simulink model "Capture_NDI"  (R2023b)
settings: Solver=FixedStepAuto  StartTime=0.0  StopTime=3500  RelTol=1e-3
values from neighbouring files (symbols this model uses):
  dim_q = robot_post_sim.n_q    [init_control_test.m]
  dim_r = robot_post_sim.dimensions.dim_r    [init_control_test.m]
  q00 = [0;0;0;1;zeros(3,1)]    [init_control_test.m]
  qm0 = q_init    [init_control_test.m]
  robot_unc_post = get_robot_unc(robot_post_sim,robot_post,E_inertia_max,E_mass_max,E_mode_max,E_mass_target_max,E_inertia_target_max)    [init_control_test.m]
  robot_unc_pre = get_robot_unc(robot_pre_sim,robot_pre,E_inertia_max,E_mass_max,E_mode_max,E_mass_target_max,E_inertia_target_max)    [init_control_test.m]
  u0_t_0 = rand(6,1)*1e-4    [init_control_test.m]
  um0 = qdot_init    [init_control_test.m]
undefined symbols (not defined in the file or in its folder): Newton, Raphson, robot_post_sim, robot_pre_sim, target_sim
libraries: SPART_Lib x1
settings Model: Creator=skraiem  LastModifiedBy=skraiem

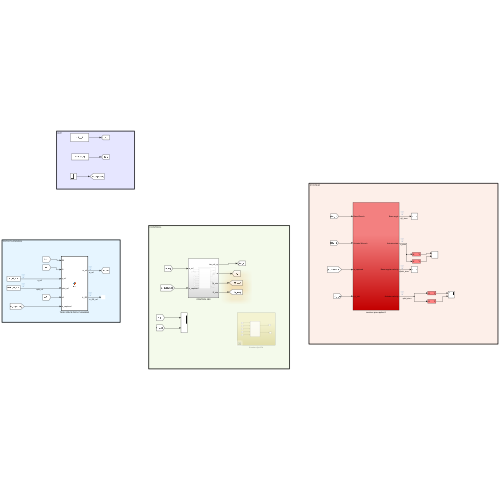
[thumbnail: Simulink's stored preview of the top-level diagram]
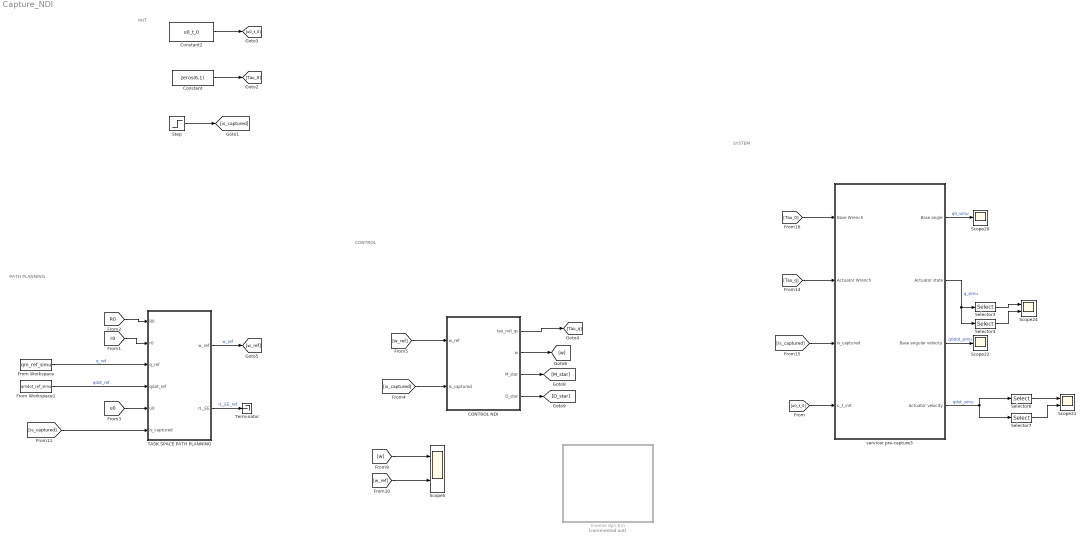
== system Capture_NDI ==
  note: SYSTEM
  note: CONTROL
  note: PATH PLANNING
  note: INIT
  CONTROL NDI : Subsystem
  Constant : Constant  Value=zeros(6,1)
  Constant2 : Constant  Value=u0_t_0
  From Workspace : FromWorkspace  VariableName=qm_ref_simu
  From Workspace1 : FromWorkspace  VariableName=qmdot_ref_simu
  Inverse dyn-Kin : Subsystem  Commented=on
  Scope20 : Scope
  Scope21 : Scope  NumInputPorts=2
  Scope22 : Scope
  Scope24 : Scope  NumInputPorts=2
  Scope5 : Scope  NumInputPorts=2
  Selector3 : Selector  IndexOptions=Index vector (dialog)  Indices=[1:dim_r]  OutputSizes=1
  Selector4 : Selector  IndexOptions=Index vector (dialog)  Indices=[dim_r+1:dim_q]  OutputSizes=1
  Selector6 : Selector  IndexOptions=Index vector (dialog)  Indices=[1:dim_r]  OutputSizes=1
  Selector7 : Selector  IndexOptions=Index vector (dialog)  Indices=[dim_r+1:dim_q]  OutputSizes=1
  Step : Step  Time=2050  SampleTime=0
  TASK SPACE PATH PLANNING : MATLAB Function  TreatAsAtomicUnit=on
  Terminator : Terminator
  servicer pre-capture3 : Subsystem
  wires:
  Step/1 -> [is_captured]
  Constant/1 -> [Tau_0]
  [Tau_0] -> servicer pre-capture3/1(Base Wrench)
  [is_captured] -> servicer pre-capture3/3(is_captured)
  servicer pre-capture3/2(Actuator state) -> Selector3/1, Selector4/1  "q_simu"
  servicer pre-capture3/4(Actuator velocity) -> Selector7/1, Selector6/1  "qdot_simu"
  servicer pre-capture3/3(Base angular velocity) -> Scope22/1  "q0dot_simu"
  servicer pre-capture3/1(Base angle) -> Scope20/1  "q0_simu"
  [u0_t_0] -> servicer pre-capture3/4(u_t_init)
  [Tau_q] -> servicer pre-capture3/2(Actuator Wrench)
  Selector3/1 -> Scope24/1
  Selector4/1 -> Scope24/2
  Selector6/1 -> Scope21/1
  Selector7/1 -> Scope21/2
  Constant2/1 -> [u0_t_0]
  From Workspace/1 -> TASK SPACE PATH PLANNING/3(q_ref)  "q_ref"
  From Workspace1/1 -> TASK SPACE PATH PLANNING/4(qdot_ref)  "qdot_ref"
  [r0] -> TASK SPACE PATH PLANNING/2(r0)
  [R0] -> TASK SPACE PATH PLANNING/1(R0)
  TASK SPACE PATH PLANNING/1(w_ref) -> [w_ref]  "w_ref"
  [u0] -> TASK SPACE PATH PLANNING/5(u0)
  [is_captured] -> CONTROL NDI/2(is_captured)
  CONTROL NDI/2(w) -> [w]
  TASK SPACE PATH PLANNING/2(rL_EE) -> Terminator/1  "rL_EE_ref"
  CONTROL NDI/1(tau_ndi_qc) -> [Tau_q]
  [w] -> Scope5/1
  [w_ref] -> Scope5/2
  [is_captured] -> TASK SPACE PATH PLANNING/6(is_captured)
  CONTROL NDI/3(M_star) -> [M_star]
  CONTROL NDI/4(D_star) -> [D_star]
  [w_ref] -> CONTROL NDI/1(w_ref)

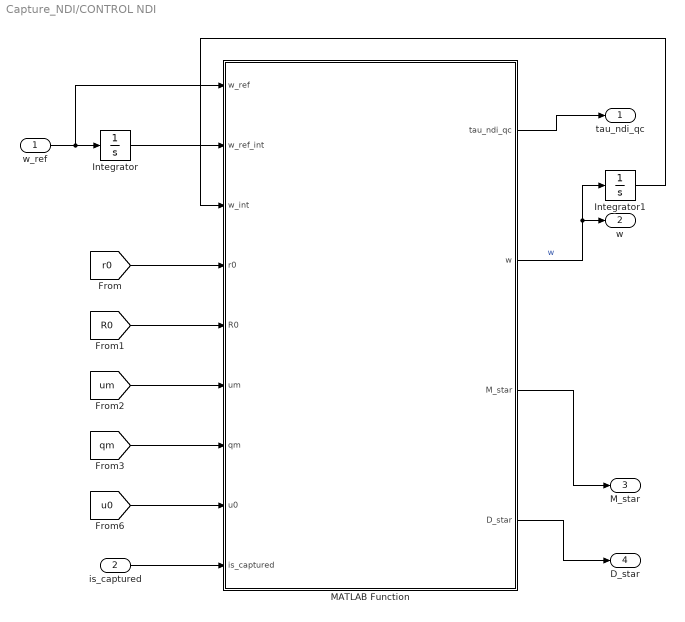
== system Capture_NDI/CONTROL NDI ==
  w_ref : Inport
  is_captured : Inport  Port=2
  Integrator : Integrator
  Integrator1 : Integrator
  MATLAB Function : MATLAB Function  TreatAsAtomicUnit=on
  tau_ndi_qc : Outport
  w : Outport  Port=2
  M_star : Outport  Port=3
  D_star : Outport  Port=4
  wires:
  w_ref/1 -> MATLAB Function/1(w_ref), Integrator/1
  [u0] -> MATLAB Function/8(u0)
  Integrator/1 -> MATLAB Function/2(w_ref_int)
  [r0] -> MATLAB Function/4(r0)
  [um] -> MATLAB Function/6(um)
  [R0] -> MATLAB Function/5(R0)
  [qm] -> MATLAB Function/7(qm)
  is_captured/1 -> MATLAB Function/9(is_captured)
  MATLAB Function/1(tau_ndi_qc) -> tau_ndi_qc/1
  MATLAB Function/2(w) -> Integrator1/1, w/1  "w"
  MATLAB Function/3(M_star) -> M_star/1
  Integrator1/1 -> MATLAB Function/3(w_int)
  MATLAB Function/4(D_star) -> D_star/1

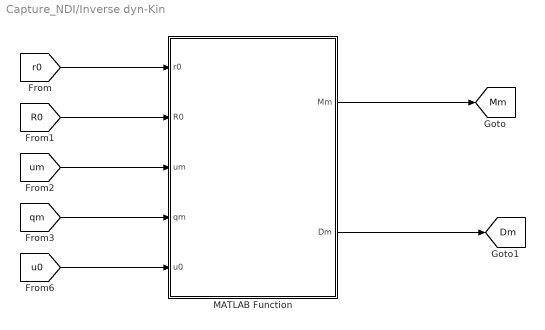
== system Capture_NDI/Inverse dyn-Kin ==
  MATLAB Function : MATLAB Function  TreatAsAtomicUnit=on
  tag scope: Dm=global, Mm=global
  wires:
  [R0] -> MATLAB Function/2(R0)
  [um] -> MATLAB Function/3(um)
  [qm] -> MATLAB Function/4(qm)
  MATLAB Function/2(Dm) -> [Dm]
  MATLAB Function/1(Mm) -> [Mm]
  [r0] -> MATLAB Function/1(r0)
  [u0] -> MATLAB Function/5(u0)

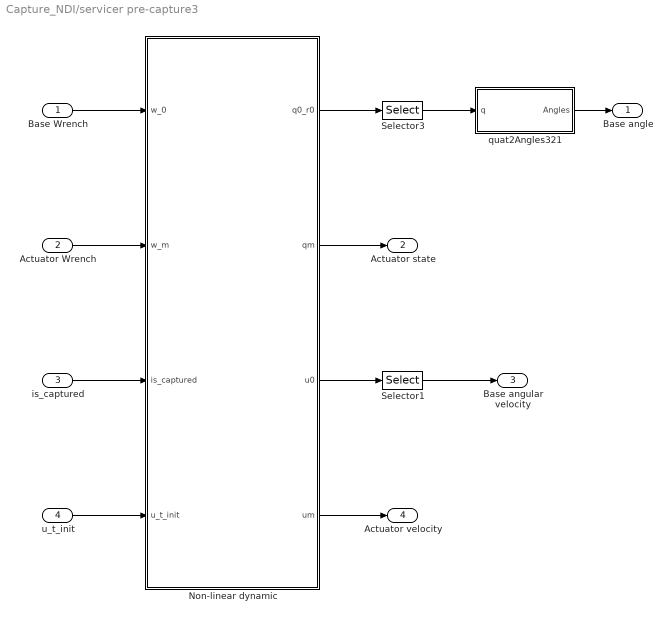
== system Capture_NDI/servicer pre-capture3 ==
  Base Wrench : Inport
  Actuator Wrench : Inport  Port=2
  is_captured : Inport  Port=3
  u_t_init : Inport  Port=4
  Non-linear dynamic : Subsystem
  Selector1 : Selector  IndexOptions=Index vector (dialog)  Indices=[1:3]  OutputSizes=1
  Selector3 : Selector  IndexOptions=Index vector (dialog)  Indices=[1:4]  OutputSizes=1
  quat2Angles321 : MATLAB Function  TreatAsAtomicUnit=on
  Base angle : Outport  VectorParamsAs1DForOutWhenUnconnected=off
  Actuator state : Outport  Port=2  VectorParamsAs1DForOutWhenUnconnected=off
  Base angular velocity : Outport  Port=3  VectorParamsAs1DForOutWhenUnconnected=off
  Actuator velocity : Outport  Port=4  VectorParamsAs1DForOutWhenUnconnected=off
  wires:
  Actuator Wrench/1 -> Non-linear dynamic/2(w_m)
  Base Wrench/1 -> Non-linear dynamic/1(w_0)
  u_t_init/1 -> Non-linear dynamic/4(u_t_init)
  is_captured/1 -> Non-linear dynamic/3(is_captured)
  Non-linear dynamic/2(qm) -> Actuator state/1
  Non-linear dynamic/1(q0_r0) -> Selector3/1
  Non-linear dynamic/3(u0) -> Selector1/1
  Non-linear dynamic/4(um) -> Actuator velocity/1
  Selector3/1 -> quat2Angles321/1(q)
  Selector1/1 -> Base angular velocity/1
  quat2Angles321/1(Angles) -> Base angle/1

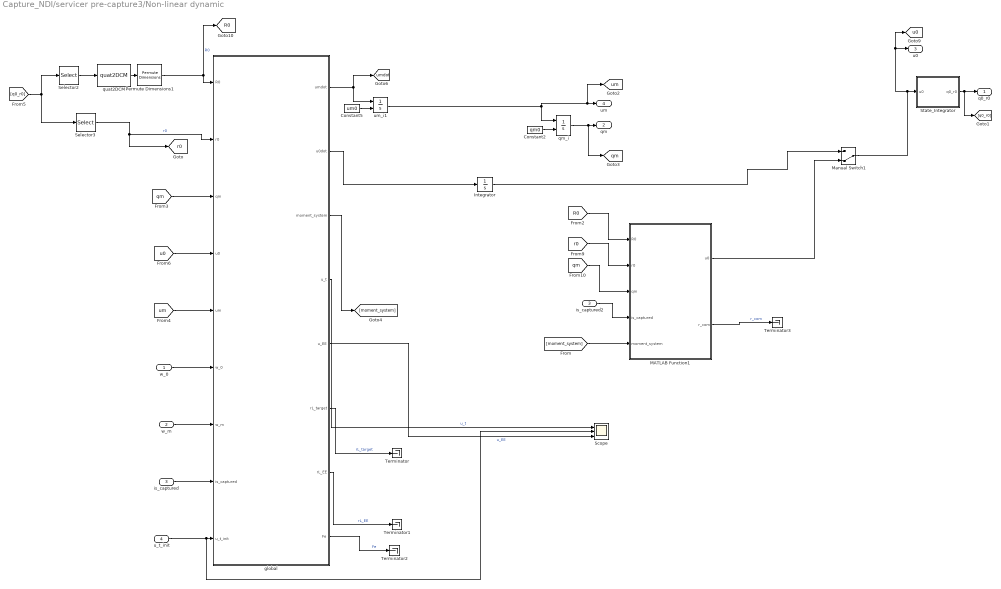
== system Capture_NDI/servicer pre-capture3/Non-linear dynamic ==
  w_0 : Inport
  w_m : Inport  Port=2
  is_captured : Inport  Port=3
  u_t_init : Inport  Port=4
  Constant2 : Constant  Value=qm0
  Constant5 : Constant  Value=um0
  Integrator : Integrator
  MATLAB Function1 : MATLAB Function  TreatAsAtomicUnit=on
  Manual Switch1 : ManualSwitch  CurrentSetting=0
  Permute Dimensions1 : PermuteDimensions
  Scope : Scope  NumInputPorts=3
  Selector2 : Selector  InputPortWidth=7  IndexOptions=Index vector (dialog)  Indices=[1:4]  OutputSizes=1
  Selector3 : Selector  InputPortWidth=7  IndexOptions=Index vector (dialog)  Indices=[5:7]  OutputSizes=1
  State_Integrator : Subsystem  AncestorBlock=SPART_Lib/Plant/State_Integrator
  Terminator{,1..3} (4 alike) : Terminator
  global : MATLAB Function  TreatAsAtomicUnit=on
  is_captured2 : InportShadow  Port=3
  qm_i : Integrator  InitialConditionSource=external
  quat2DCM : SPART_Lib/Components/Matrices/quat2DCM  SystemSampleTime=-1  VariantActivationTime=update diagram  AllowFlexibleInterface=on  Latency=0  AutoFrameSizeCalculation=off
  um_i1 : Integrator  InitialConditionSource=external
  q0_r0 : Outport  VectorParamsAs1DForOutWhenUnconnected=off
  qm : Outport  Port=2  VectorParamsAs1DForOutWhenUnconnected=off
  u0 : Outport  Port=3  VectorParamsAs1DForOutWhenUnconnected=off
  um : Outport  Port=4  VectorParamsAs1DForOutWhenUnconnected=off
  tag scope: R0=global, qm=global, r0=global, u0=global, um=global, umdot=global
  wires:
  Selector2/1 -> quat2DCM/1
  Permute Dimensions1/1 -> [R0], global/1(R0)  "R0"
  [qm] -> global/3(qm)
  w_0/1 -> global/6(w_0)
  [um] -> global/5(um)
  qm_i/1 -> [qm], qm/1
  [q0_r0] -> Selector3/1, Selector2/1
  [u0] -> global/4(u0)
  Selector3/1 -> [r0], global/2(r0)  "r0"
  w_m/1 -> global/7(w_m)
  quat2DCM/1 -> Permute Dimensions1/1
  Constant2/1 -> qm_i/2
  um_i1/1 -> qm_i/1, [um], um/1
  State_Integrator/1(q0_r0) -> [q0_r0], q0_r0/1
  Constant5/1 -> um_i1/2
  global/1(umdot) -> um_i1/1, [umdot]
  is_captured/1 -> global/8(is_captured)
  Manual Switch1/1 -> [u0], u0/1, State_Integrator/1(u0)
  global/2(u0dot) -> Integrator/1
  Integrator/1 -> Manual Switch1/1
  u_t_init/1 -> Scope/2, global/9(u_t_init)
  MATLAB Function1/1(u0) -> Manual Switch1/2
  is_captured2/1 -> MATLAB Function1/4(is_captured)
  [qm] -> MATLAB Function1/3(qm)
  [r0] -> MATLAB Function1/2(r0)
  [R0] -> MATLAB Function1/1(R0)
  global/3(moment_system) -> [moment_system]
  global/4(u_t) -> Scope/1  "u_t"
  global/5(u_EE) -> Scope/3  "u_EE"
  [moment_system] -> MATLAB Function1/5(moment_system)
  global/6(rL_target) -> Terminator/1  "rL_target"
  global/7(rL_EE) -> Terminator1/1  "rL_EE"
  global/8(Fe) -> Terminator2/1  "Fe"
  MATLAB Function1/2(r_com) -> Terminator3/1  "r_com"

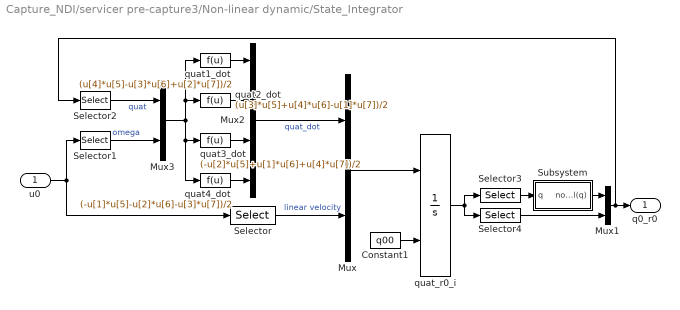
== system Capture_NDI/servicer pre-capture3/Non-linear dynamic/State_Integrator ==
  u0 : Inport
  Constant1 : Constant  Value=q00
  Mux : Mux  Inputs=2
  Mux1 : Mux  Inputs=2
  Mux2 : Mux
  Mux3 : Mux  Inputs=2
  Selector : Selector  InputPortWidth=6  IndexOptions=Index vector (dialog)  Indices=[4:6]  OutputSizes=1
  Selector1 : Selector  InputPortWidth=6  IndexOptions=Index vector (dialog)  Indices=[1:3]  OutputSizes=1
  Selector2 : Selector  InputPortWidth=7  IndexOptions=Index vector (dialog)  Indices=[1:4]  OutputSizes=1
  Selector3 : Selector  InputPortWidth=7  IndexOptions=Index vector (dialog)  Indices=[1:4]  OutputSizes=1
  Selector4 : Selector  InputPortWidth=7  IndexOptions=Index vector (dialog)  Indices=[5:7]  OutputSizes=1
  Subsystem : Subsystem
  quat1_dot : Fcn  Expr=(u[4]*u[5]-u[3]*u[6]+u[2]*u[7])/2
  quat2_dot : Fcn  Expr=(u[3]*u[5]+u[4]*u[6]-u[1]*u[7])/2
  quat3_dot : Fcn  Expr=(-u[2]*u[5]+u[1]*u[6]+u[4]*u[7])/2
  quat4_dot : Fcn  Expr=(-u[1]*u[5]-u[2]*u[6]-u[3]*u[7])/2
  quat_r0_i : Integrator  InitialConditionSource=external
  q0_r0 : Outport  VectorParamsAs1DForOutWhenUnconnected=off
  wires:
  Selector2/1 -> Mux3/1  "quat"
  quat4_dot/1 -> Mux2/4
  quat3_dot/1 -> Mux2/3
  quat2_dot/1 -> Mux2/2
  quat1_dot/1 -> Mux2/1
  Mux3/1 -> quat2_dot/1, quat1_dot/1, quat3_dot/1, quat4_dot/1
  Selector4/1 -> Mux1/2
  Selector3/1 -> Subsystem/1(q)
  quat_r0_i/1 -> Selector3/1, Selector4/1
  Subsystem/1(normal(q)) -> Mux1/1
  Selector1/1 -> Mux3/2  "omega"
  Mux1/1 -> q0_r0/1, Selector2/1
  u0/1 -> Selector1/1, Selector/1
  Selector/1 -> Mux/2  "linear velocity"
  Mux2/1 -> Mux/1  "quat_dot"
  Mux/1 -> quat_r0_i/1
  Constant1/1 -> quat_r0_i/2

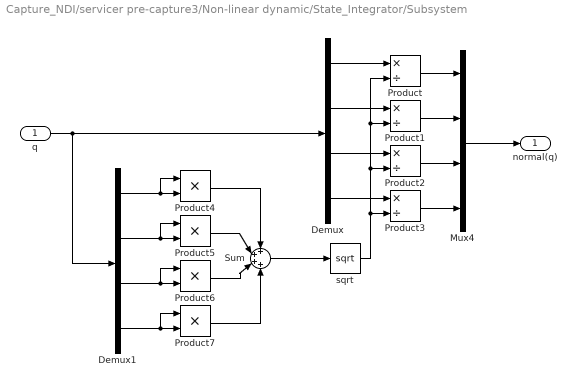
== system Capture_NDI/servicer pre-capture3/Non-linear dynamic/State_Integrator/Subsystem ==
  q : Inport
  Demux : Demux
  Demux1 : Demux
  Mux4 : Mux
  Product{,1..3} (4 alike) : Product  Inputs=*/
  Product{4..7} (4 alike) : Product
  Sum : Sum  Inputs=4
  sqrt : Sqrt  AlgorithmType=Newton-Raphson
  normal(q) : Outport  VectorParamsAs1DForOutWhenUnconnected=off
  wires:
  q/1 -> Demux/1, Demux1/1
  Sum/1 -> sqrt/1
  Product4/1 -> Sum/1
  Product5/1 -> Sum/2
  Product6/1 -> Sum/3
  Product7/1 -> Sum/4
  Demux1/1 -> Product4/2, Product4/1
  Demux1/2 -> Product5/2, Product5/1
  Demux1/3 -> Product6/2, Product6/1
  Demux1/4 -> Product7/2, Product7/1
  Demux/4 -> Product3/1
  Demux/2 -> Product1/1
  Demux/1 -> Product/1
  Demux/3 -> Product2/1
  Mux4/1 -> normal(q)/1
  sqrt/1 -> Product1/2, Product/2, Product2/2, Product3/2
  Product/1 -> Mux4/1
  Product1/1 -> Mux4/2
  Product2/1 -> Mux4/3
  Product3/1 -> Mux4/4

== matlab function Capture_NDI/Inverse dyn-Kin/MATLAB Function ==
  data: r0 input; R0 input; um input; qm input; u0 input; Mm output; Dm output; robot_unc parameter
function [Mm,Dm]  = fcn(r0,R0,um,qm,u0,robot_unc)





%--- System_dimension ---%
dim_0 = 6;
dim_m = robot_unc.n_q;
dim_f = robot_unc.flexs.nb_mode; 

%--- Kinematics ---%
%Kinematics
[~,RL,rJ,rL,e,g]    =   Kinematics(R0,r0,qm,robot_unc);

%Diferential Kinematics
[Bij,Bi0,P0,pm]     =   DiffKinematics(R0,r0,rL,e,g,robot_unc);
%Velocities
[t0,tL]             =   Velocities(Bij,Bi0,P0,pm,u0,um,robot_unc);
%Jacobian of the flexible link
[Jf0, Jfm]          =   Jacob_flex(rJ,r0,rL,P0,pm,robot_unc);
[Jf0dot, Jfmdot]    =   Jacobdot_flex(rJ,r0,t0,rL,tL,P0,pm,Jf0, Jfm,u0,um,robot_unc);

%--- Dynamics ---%
%Inertias in inertial frames
[I0,Im]             =   I_I(R0,RL,robot_unc);
%Mass Composite Body matrix
[M0_tilde,Mm_tilde] =   MCB(I0,Im,Bij,Bi0,robot_unc);
%Generalized Inertia matrix
[H0,H0m,Hm]         =   GIM(M0_tilde,Mm_tilde,Bij,Bi0,P0,pm,robot_unc);
[Hf0, Hfm, Hf]      =   GIM_flex(RL,Jf0, Jfm,robot_unc);
%Generalized Convective Inertia matrix
[C0, C0m, Cm0, Cm]  =   CIM(t0,tL,I0,Im,M0_tilde,Mm_tilde,Bij,Bi0,P0,pm,robot_unc);

[Cf0, Cfm, Cf]      =   CIM_flex(RL,Jf0dot, Jfmdot,robot_unc);
%Stifness matrix of flexible links
[Kf]                =   Stif_flex(robot_unc);

Mm =...
    [H0 H0m Hf0' ;...
    H0m' Hm Hfm';...
    Hf0 Hfm Hf];

Dm =...
    [C0 C0m Cf0' ;...
    Cm0 Cm Cfm';...
    Cf0 Cfm Cf];

== matlab function Capture_NDI/CONTROL NDI/MATLAB Function ==
  data: w_ref input; w_ref_int input; w_int input; r0 input; R0 input; um input; qm input; u0 input; tau_ndi_qc output; robot_unc_pre parameter; robot_unc_post parameter; is_captured input; w output; M_star output; D_star output
function [tau_ndi_qc,w,M_star,D_star]= fcn(w_ref,w_ref_int,w_int,r0,R0,um,qm,u0,robot_unc_pre, robot_unc_post, is_captured)
    
    %-- Dimensions --%
    dim_0 = 6;
    dim_q = robot_unc_pre.n_q;
    dim_r = robot_unc_pre.dimensions.dim_r;
    dim_m = robot_unc_pre.dimensions.dim_m;


    if is_captured 

         %--- Kinematics ---%
        %Kinematics
        [~,RL,rJ,rL,e,g]    =   Kinematics(R0,r0,qm,robot_unc_post);
        
        %Diferential Kinematics
        [Bij,Bi0,P0,pm]     =   DiffKinematics(R0,r0,rL,e,g,robot_unc_post);
        %Velocities
        [t0,tL]             =   Velocities(Bij,Bi0,P0,pm,u0,um,robot_unc_post);
        
        %--- Dynamics ---%
        %Inertias in inertial frames
        [I0,Im]             =   I_I(R0,RL,robot_unc_post);
        %Mass Composite Body matrix
        [M0_tilde,Mm_tilde] =   MCB(I0,Im,Bij,Bi0,robot_unc_post);
        %Generalized Inertia matrix
        [H0,H0q,Hq]         =   GIM(M0_tilde,Mm_tilde,Bij,Bi0,P0,pm,robot_unc_post);
        %Generalized Convective Inertia matrix
        [C0, C0q, Cq0, Cq]  =   CIM(t0,tL,I0,Im,M0_tilde,Mm_tilde,Bij,Bi0,P0,pm,robot_unc_post);
        u_EE = tL(:,robot_unc_post.id_EE);
        Mm =[H0 H0q ;...
            H0q' Hq];
        
        Dm =[C0 C0q ;
            Cq0 Cq];

        [J0EE, JmEE]        =   Jacob(rL(:,robot_unc_post.id_EE),r0,rL,P0,pm,robot_unc_post.id_EE,robot_unc_post);
        [J0EEdot, JmEEdot]  =   Jacobdot(rL(:,robot_unc_post.id_EE),u_EE,r0,u0,rL,tL,P0,pm,robot_unc_post.id_EE,robot_unc_post);


        [I0_dot,I_Idot] = I_I_dot(R0, t0, RL,tL,robot_unc_post);
        [N] = NOC(r0,rL,P0,pm,robot_unc_post);
        [Ndot] = NOCdot(r0,t0,rL,tL,P0,pm,robot_unc_post);
        [H0_dot, H0q_dot, Hq_dot]=GIM_NOCdot_parsed(N, Ndot,I0,Im,I0_dot,I_Idot,robot_unc_post);

        % [H0_dot, H0q_dot, Hq_dot ] = H_dot_Lagrange(Im,Bi0,P0,R0,pm,r0,t0,rL,tL,RL,robot_unc_post);
    
    else 


        %--- Kinematics ---%
        %Kinematics
        [~,RL,rJ,rL,e,g]    =   Kinematics(R0,r0,qm,robot_unc_pre);
        
        %Diferential Kinematics
        [Bij,Bi0,P0,pm]     =   DiffKinematics(R0,r0,rL,e,g,robot_unc_pre);
        %Velocities
        [t0,tL]             =   Velocities(Bij,Bi0,P0,pm,u0,um,robot_unc_pre);
        
        %--- Dynamics ---%
        %Inertias in inertial frames
        [I0,Im]             =   I_I(R0,RL,robot_unc_pre);
        %Mass Composite Body matrix
        [M0_tilde,Mm_tilde] =   MCB(I0,Im,Bij,Bi0,robot_unc_pre);
        %Generalized Inertia matrix
        [H0,H0q,Hq]         =   GIM(M0_tilde,Mm_tilde,Bij,Bi0,P0,pm,robot_unc_pre);
        %Generalized Convective Inertia matrix
        [C0, C0q, Cq0, Cq]  =   CIM(t0,tL,I0,Im,M0_tilde,Mm_tilde,Bij,Bi0,P0,pm,robot_unc_pre);
        u_EE = tL(:,robot_unc_pre.id_EE);
        
        Mm =[H0 H0q ;...
            H0q' Hq];
        
        Dm =[C0 C0q ;
            Cq0 Cq];

        [J0EE, JmEE]      =   Jacob(rL(:,robot_unc_pre.id_EE),r0,rL,P0,pm,robot_unc_pre.id_EE,robot_unc_pre);
        [J0EEdot, JmEEdot]  =   Jacobdot(rL(:,robot_unc_pre.id_EE),u_EE,r0,u0,rL,tL,P0,pm,robot_unc_pre.id_EE,robot_unc_pre);
        
        [I0_dot,I_Idot] = I_I_dot(R0, t0, RL,tL,robot_unc_pre);
        [N] = NOC(r0,rL,P0,pm,robot_unc_pre);
        [Ndot] = NOCdot(r0,t0,rL,tL,P0,pm,robot_unc_pre);
        [H0_dot, H0q_dot, Hq_dot]=GIM_NOCdot_parsed(N, Ndot,I0,Im,I0_dot,I_Idot,robot_unc_pre);

        % [H0_dot, H0q_dot, Hq_dot ] = H_dot_Lagrange(Im,Bi0,P0,R0,pm,r0,t0,rL,tL,RL,robot_unc_pre);
        
        
    end



    %-- Rigid task Space --%
    %tasks: w0, tee
    
    Hw  = H0(1:3,1:3);
    HwL = H0(1:3,4:6);
    HL  = H0(4:6,4:6);
    Hwq = H0q(1:3,:);
    HLq = H0q(4:6,:);
    
    Hwdot  = H0_dot(1:3,1:3);
    HwLdot = H0_dot(1:3,4:6);
    HLdot  = H0_dot(4:6,4:6);
    Hwqdot = H0q_dot(1:3,:);
    HLqdot = H0q_dot(4:6,:);

    invHL = inv(HL);
    Jomega = -(Hw-HwL*invHL*HwL')*(Hwq-HwL*invHL*HLq);
    % Jomega_dot = Hwdot*Hwq + Hw*Hwqdot-HwLdot*invHL*HwL'*Hwq-HwL*inv(HLdot)*HwL'*Hwq-HwL*invHL*HwLdot'*Hwq-HwL*invHL*HwL'*Hwqdot...
    %             -Hwdot*HwL*invHL*HLq-Hw*HwLdot*invHL*HLq-Hw*HwL*inv(HLdot)*HLq-Hw*HwL*invHL*HLqdot...
    %             +HwLdot*invHL*HwL'*HwL*invHL*HLq+HwL*inv(HLdot)*HwL'*HwL*invHL*HLq+HwL*invHL*HwLdot'*HwL*invHL*HLq+HwL*invHL*HwL'*HwLdot*invHL*HLq...
    %             +HwL*invHL*HwL'*HwL*inv(HLdot)*HLq+HwL*invHL*HwL'*HwL*invHL*HLqdot; 
    % Jomega_dot = Hwdot*Hwq + Hw*Hwqdot-HwLdot*invHL*HwL'*Hwq-HwL*inv(HLdot)*HwL'*Hwq-HwL*invHL*HwLdot'*Hwq-HwL*invHL*HwL'*Hwqdot...
    %             -Hwdot*HwL*invHL*HLq-Hw*HwLdot*invHL*HLq-Hw*HwL*inv(HLdot)*HLq-Hw*HwL*invHL*HLqdot...
    %             +HwLdot*invHL*HwL'*HwL*invHL*HLq+HwL*inv(HLdot)*HwL'*HwL*invHL*HLq+HwL*invHL*HwLdot'*HwL*invHL*HLq+HwL*invHL*HwL'*HwLdot*invHL*HLq...
    %             +HwL*invHL*HwL'*HwL*inv(HLdot)*HLq+HwL*invHL*HwL'*HwL*invHL*HLqdot; 

    Jomega_dot = Hwdot*Hwq + Hw*Hwqdot-HwLdot*invHL*HwL'*Hwq-HwL*invHL*HwLdot'*Hwq-HwL*invHL*HwL'*Hwqdot...
                -Hwdot*HwL*invHL*HLq-Hw*HwLdot*invHL*HLq-Hw*HwL*invHL*HLqdot...
                +HwLdot*invHL*HwL'*HwL*invHL*HLq+HwL*invHL*HwLdot'*HwL*invHL*HLq+HwL*invHL*HwL'*HwLdot*invHL*HLq...
                +HwL*invHL*HwL'*HwL*invHL*HLqdot; 

    JEE_star = JmEE-J0EE*inv(H0)*H0q;
    JEE_star_dot =JmEEdot-J0EEdot*inv(H0)*H0q-J0EE*inv(H0_dot)*H0q-J0EE*inv(H0)*H0q_dot;
    J = [Jomega;JEE_star];
    Jdot = [Jomega_dot;JEE_star_dot];


%     invH0 = inv(H0);
%     M_star = Hq-H0q'*invH0*H0q;
%     D_star = Cq -(Cq0-H0q'*invH0*C0)*invH0*H0q -H0q'*invH0*C0q;
%     Dh_star = (Cq0-H0q'*invH0*C0)*invH0;
% 
% 
% 
%     %if initial momentum null
%     Mq_diamond = Hq -H0q.'*invH0*H0q;
% %     Dq_diamond = Cq - Cq0*invH0*C0q + H0q.'*invH0*C0*invH0*H0q;
%     %else
%     Dq_diamond  = Cq - H0q.'*invH0*C0q;
%     Dq0_diamond = Cq0 - H0q.'*invH0*C0;


    %%--Dyn diamond --%%
    invH0 = inv(H0);
    M_diamond = Hq -H0q'*invH0*H0q;
    D_diamond = Cq -(Cq0-H0q'*invH0*C0)*invH0*H0q -H0q'*invH0*C0q;
    
    %%--Dyn star --%%
    M_star = M_diamond*inv(J);
    D_star = D_diamond;%-M_diamond*inv(J)*Jdot;
    
    
    w1 = u0(1:3,1);
    w2 = u_EE;
    w = [w1;w2];



M_star_inv = inv(M_star);

tau_ndi_qc =M_star* robot_unc_pre.control.Kp*(w_ref-w) +M_star* robot_unc_pre.control.Kv*(w_ref_int-w_int) +D_star*w;
% tau_ndi_qc =M_star* robot_unc_pre.control.Kp*(w_ref-w)  +D_star*w;

== matlab function Capture_NDI/TASK SPACE PATH PLANNING ==
  data: R0 input; r0 input; q_ref input; qdot_ref input; u0 input; is_captured input; w_ref output; robot_pre_sim parameter; rL_EE output
function [w_ref,rL_EE]= fcn(R0,r0,q_ref,qdot_ref,u0, is_captured,robot_pre_sim)

qm = [zeros(robot_pre_sim.dimensions.dim_r,1);q_ref];
qmdot = [0*150*ones(robot_pre_sim.dimensions.dim_r,1);qdot_ref];



[~,RL,~,rL,e,g]    =   Kinematics(R0,r0,qm,robot_pre_sim);
%Diferential Kinematics
[Bij,Bi0,P0,pm]     =   DiffKinematics(R0,r0,rL,e,g,robot_pre_sim);
[t0,tL]             =   Velocities(Bij,Bi0,P0,pm,u0,qmdot,robot_pre_sim);
u_EE = tL(:,robot_pre_sim.id_EE);
rL_EE       = rL(:,robot_pre_sim.id_EE);

 %--- Dynamics ---%
%Inertias in inertial frames
[I0,Im]             =   I_I(R0,RL,robot_pre_sim);
%Mass Composite Body matrix
[M0_tilde,Mm_tilde] =   MCB(I0,Im,Bij,Bi0,robot_pre_sim);
%Generalized Inertia matrix
[H0,H0q,Hq]         =   GIM(M0_tilde,Mm_tilde,Bij,Bi0,P0,pm,robot_pre_sim);


[J0EE, JmEE]      =   Jacob(rL(:,robot_pre_sim.id_EE),r0,rL,P0,pm,robot_pre_sim.id_EE,robot_pre_sim);

w1 = zeros(3,1);
w1 = -inv(H0)*H0q*qmdot;
w1 = 0*w1(1:3,1);
w2 = J0EE*u0+JmEE*qmdot;
w2 = u_EE;


if is_captured
    w2 = 0*u_EE;
else
    w2 = u_EE;
end

w_ref = [w1;w2];

== matlab function Capture_NDI/servicer pre-capture3/Non-linear dynamic/MATLAB Function1 ==
  data: R0 input; u0 output; r0 input; qm input; is_captured input; moment_system input; robot_post_sim parameter; robot_pre_sim parameter; r_com output
function [u0,r_com] = ddX(R0,r0,qm,is_captured,moment_system,robot_post_sim,robot_pre_sim)

% :inputs:
%   * R0 -- Rotation matrix from the base-link CCS to the inertial CCS -- [3x3].
%   * r0 -- Position of the base-link center-of-mass with respect to the origin of the inertial frame,
%projected in the inertial CCS -- [3x1].
%   * qm -- Displacements of the active joints -- [n_qx1].
%   * eta -- Modal
%   * u0 -- Base-link velocities [\omega,rdot]. The angular velocity is projected in the body-fixed CCS,
%while the linear velocity is projected in the inertial CCS -- [6x1].
%   * um -- Joint velocities -- [n_qx1].
%   * robot -- Robot model (see :doc:`/Tutorial_Robot`).

%--- System_dimension ---%
dim_0 = 6;



if is_captured
    robot_sim = robot_post_sim;
    %--- Kinematics ---%
    %Kinematics
    [~,RL,~,rL,e,g]    =   Kinematics(R0,r0,qm,robot_sim);
    
    %Diferential Kinematics
    [Bij,Bi0,P0,pm]     =   DiffKinematics(R0,r0,rL,e,g,robot_sim);
    %Velocities
    %Inertias in inertial frames
    [I0,Im]             =   I_I(R0,RL,robot_sim);
    %Mass Composite Body matrix
    [M0_tilde,Mm_tilde] =   MCB(I0,Im,Bij,Bi0,robot_sim);
    %Generalized Inertia matrix
    [H0,H0m,~]         =   GIM(M0_tilde,Mm_tilde,Bij,Bi0,P0,pm,robot_sim);
    %u0=-inv(H0)*H0m*um +inv(H0)*moment_target_init;
    u0 = -inv(H0)*moment_system;
    r_com =Center_of_Mass(r0,rL,robot_sim);


else
    robot_sim = robot_pre_sim;
     %--- Kinematics ---%
    %Kinematics
    [~,RL,~,rL,e,g]    =   Kinematics(R0,r0,qm,robot_sim);
    
    %Diferential Kinematics
    [Bij,Bi0,P0,pm]     =   DiffKinematics(R0,r0,rL,e,g,robot_sim);
    %Velocities
    %Inertias in inertial frames
    [I0,Im]             =   I_I(R0,RL,robot_sim);
    %Mass Composite Body matrix
    [M0_tilde,Mm_tilde] =   MCB(I0,Im,Bij,Bi0,robot_sim);
    %Generalized Inertia matrix
    [H0,H0m,~]         =   GIM(M0_tilde,Mm_tilde,Bij,Bi0,P0,pm,robot_sim);
    %u0=-inv(H0)*H0m*um;
    u0 = -inv(H0)*moment_system;
    r_com =Center_of_Mass(r0,rL,robot_sim);
    
end

== matlab function Capture_NDI/servicer pre-capture3/Non-linear dynamic/global ==
  data: umdot output; u0dot output; R0 input; r0 input; qm input; u0 input; um input; w_0 input; w_m input; is_captured input; u_t_init input; robot_pre_sim parameter; target_sim parameter; moment_system output; u_t output; u_EE output; rL_target output; rL_EE output; Fe output
function [umdot,u0dot,moment_system,u_t,u_EE,rL_target,rL_EE,Fe] = ddX(R0,r0,qm,u0,um,w_0,w_m,is_captured,u_t_init,robot_pre_sim,target_sim)

% :inputs:
%   * R0 -- Rotation matrix from the base-link CCS to the inertial CCS -- [3x3].
%   * r0 -- Position of the base-link center-of-mass with respect to the origin of the inertial frame,
%projected in the inertial CCS -- [3x1].
%   * qm -- Displacements of the active joints -- [n_qx1].
%   * eta -- Modal
%   * u0 -- Base-link velocities [\omega,rdot]. The angular velocity is projected in the body-fixed CCS,
%while the linear velocity is projected in the inertial CCS -- [6x1].
%   * um -- Joint velocities -- [n_qx1].
%   * robot -- Robot model (see :doc:`/Tutorial_Robot`).

%--- System_dimension ---%
dim_0 = 6;
dim_m = robot_pre_sim.n_q;
dim_r = robot_pre_sim.dimensions.dim_r;

%-- memory allocation --%
ddX = zeros(dim_0+dim_m,1);
u0dot = zeros(dim_0,1);
umdot = zeros(dim_m,1);


%-- SERVICER --% 
%--- Kinematics ---%
%Kinematics
[~,RL,~,rL,e,g]    =   Kinematics(R0,r0,qm,robot_pre_sim);

%Diferential Kinematics
[Bij,Bi0,P0,pm]     =   DiffKinematics(R0,r0,rL,e,g,robot_pre_sim);
%Velocities
[t0,tL]             =   Velocities(Bij,Bi0,P0,pm,u0,um,robot_pre_sim);

%--- Dynamics ---%
%Inertias in inertial frames
[I0,Im]             =   I_I(R0,RL,robot_pre_sim);
%Mass Composite Body matrix
[M0_tilde,Mm_tilde] =   MCB(I0,Im,Bij,Bi0,robot_pre_sim);
%Generalized Inertia matrix
[H0,H0m,Hm]         =   GIM(M0_tilde,Mm_tilde,Bij,Bi0,P0,pm,robot_pre_sim);
%Generalized Convective Inertia matrix
[C0, C0m, Cm0, Cm]  =   CIM(t0,tL,I0,Im,M0_tilde,Mm_tilde,Bij,Bi0,P0,pm,robot_pre_sim);

H =[H0 H0m  ;...
    H0m' Hm];

C =[C0 C0m ;...
    Cm0 Cm ];


moment_servicer = H0*u0+H0m*um;
u_EE= tL(:,robot_pre_sim.id_EE);

%-- TARGET --%
%--- Kinematics ---%
%Kinematics
[~,RL,~,rL,e,g]    =   Kinematics(R0,r0,qm,target_sim);

%Diferential Kinematics
[Bij,Bi0,P0,pm]     =   DiffKinematics(R0,r0,rL,e,g,target_sim);

%--- Dynamics ---%
%Inertias in inertial frames
[I0,Im]             =   I_I(R0,RL,target_sim);
%Mass Composite Body matrix
[M0_tilde,Mm_tilde] =   MCB(I0,Im,Bij,Bi0,target_sim);
%Generalized Inertia matrix
[H0_t,~,~]         =   GIM(M0_tilde,Mm_tilde,Bij,Bi0,P0,pm,target_sim);
[C0_t, ~, ~, ~]    =   CIM(t0,tL,I0,Im,M0_tilde,Mm_tilde,Bij,Bi0,P0,pm,target_sim);

rL_target = rL(:,target_sim.id_target);
rL_EE     = rL(:,target_sim.id_EE);

if is_captured 
    [Jt0, Jtm]      =   Jacob(rL(:,target_sim.id_target),r0,rL,P0,pm,target_sim.id_target,target_sim);
    u_t = Jt0*u0+Jtm*um;
    [Jt0dot, Jtmdot]      =   Jacobdot(rL(:,target_sim.id_target),u_t,r0,u0,rL,tL,P0,pm,target_sim.id_target,target_sim);
    udot_t = Jt0*u0dot+Jtm*umdot + Jt0dot*u0+Jtmdot*um;
    J = [Jt0 Jtm];
    Jdot = [Jt0dot Jtmdot];
    B_tEE = Bij(:,:,target_sim.id_target,target_sim.id_EE);
    
    H_star = H +J'*inv(B_tEE')*H0_t*J;
    C_star = C +J'*inv(B_tEE')*C0_t*J+J'*inv(B_tEE')*H0_t*Jdot;

    iMm = inv(H_star);
    ddX = iMm * [w_0;w_m]- iMm * C_star * [u0;um];
    u0dot = ddX(1:dim_0,1);
    umdot= ddX(dim_0+1:dim_0+dim_m,1);

    moment_t = H0_t *u_t_init;
    moment_system = moment_servicer+moment_t;

    Fe = -inv(B_tEE)'*(H0_t*udot_t+C0_t*u_t);

else 
    moment_t = H0_t *u_t_init;
    u_t = u_t_init;

    iMm = inv(H);
    ddX = iMm * [w_0;w_m]- iMm * C * [u0;um];
    u0dot = ddX(1:dim_0,1);
    umdot= ddX(dim_0+1:dim_0+dim_m,1);

    moment_system = H0*u0+H0m*um;
    B_tEE = Bij(:,:,target_sim.id_target,target_sim.id_EE);
    Fe = -inv(B_tEE)'*(C0_t*u_t);

    
    
end

== matlab function Capture_NDI/servicer pre-capture3/quat2Angles321 ==
  data: q input; Angles output
function Angles = quat2Angles321(q)
%Convert the quaternion to Euler angles (321 sequence), x-phi, y-theta, z-psi.
%
%Uses the functions under the Utilities folder


Angles = quat_Angles321(q);

end
